simulink model "ES101A_DiagcMgr"  (R2013b)
settings: Solver=ode45  StartTime=0.0  StopTime=0.44  RelTol=1e-3
values from neighbouring files (symbols this model uses):
  BrdgVltg = DataDict.IpSignal    [ES101A_DiagcMgr_DataDict.m]
  DEM_CLEAR_PENDING = DataDict.Constant    [ES101A_DiagcMgr_DataDict.m]
  DEM_DTC_GROUP_ALL_DTCS = DataDict.Constant    [ES101A_DiagcMgr_DataDict.m]
  DFTAGICNTR_CNT_U08 = DataDict.Constant    [ES101A_DiagcMgr_DataDict.m]
  DIAGCMGR_NTCINFOSTSTESTFAILD_CNT_U08 = DataDict.Constant    [ES101A_DiagcMgr_DataDict.m]
  DIAGCMGR_NTCINFOSTSTESTFAILDTHISIGNCYC_CNT_U08 = DataDict.Constant    [ES101A_DiagcMgr_DataDict.m]
  DIAGCMGR_NTCINFOSTSTESTNOTCMPLTHISIGNCYC_CNT_U08 = DataDict.Constant    [ES101A_DiagcMgr_DataDict.m]
  DiagcMgrFltResp = DataDict.Calibration    [ES101A_DiagcMgr_DataDict.m]
  DiagcMgrNtcFltAry = DataDict.NVM    [ES101A_DiagcMgr_DataDict.m]
  DIAGCSTSCTRLDSHTDWNFLTPRSNT_CNT_U16 = DataDict.Constant    [ES101A_DiagcMgr_DataDict.m]
  DIAGCSTSDFTHWAG_CNT_U16 = DataDict.Constant    [ES101A_DiagcMgr_DataDict.m]
  DIAGCSTSDFTHWAGSERLCOMEXPRTVAL_CNT_U16 = DataDict.Constant    [ES101A_DiagcMgr_DataDict.m]
  DIAGCSTSDFTVEHSPD_CNT_U16 = DataDict.Constant    [ES101A_DiagcMgr_DataDict.m]
  DIAGCSTSININVAL_CNT_U16 = DataDict.Constant    [ES101A_DiagcMgr_DataDict.m]
  DIAGCSTSIVTR1INACTV_CNT_U16 = DataDict.Constant    [ES101A_DiagcMgr_DataDict.m]
  DIAGCSTSIVTR2INACTV_CNT_U16 = DataDict.Constant    [ES101A_DiagcMgr_DataDict.m]
  DIAGCSTSLIMDTPRFMNC_CNT_U16 = DataDict.Constant    [ES101A_DiagcMgr_DataDict.m]
  DIAGCSTSRAMPTOZEROFLTPRSNT_CNT_U16 = DataDict.Constant    [ES101A_DiagcMgr_DataDict.m]
  DIAGCSTSWHLIMBREJCTNDI_CNT_U16 = DataDict.Constant    [ES101A_DiagcMgr_DataDict.m]
  DTCIDXSTSFAIL_CNT_U08 = DataDict.Constant    [ES101A_DiagcMgr_DataDict.m]
  DTCIDXSTSNONTC_CNT_U08 = DataDict.Constant    [ES101A_DiagcMgr_DataDict.m]
  DTCIDXSTSNORES_CNT_U08 = DataDict.Constant    [ES101A_DiagcMgr_DataDict.m]
  DTCIDXSTSPASS_CNT_U08 = DataDict.Constant    [ES101A_DiagcMgr_DataDict.m]
  DTCIDXSTSUPDCFMD_CNT_U08 = DataDict.Constant    [ES101A_DiagcMgr_DataDict.m]
  ELECGLBPRM_IVTRCNT_CNT_U08 = DataDict.ConfigParam    [ES101A_DiagcMgr_DataDict.m]
  FLTINJ_DIAGCMGR_DIAGCSTSIVTR1INACTV = DataDict.Constant    [ES101A_DiagcMgr_DataDict.m]
  FLTINJ_DIAGCMGR_DIAGCSTSIVTR2INACTV = DataDict.Constant    [ES101A_DiagcMgr_DataDict.m]
  HwTq = DataDict.IpSignal    [ES101A_DiagcMgr_DataDict.m]
  IgnCntr = DataDict.IpSignal    [ES101A_DiagcMgr_DataDict.m]
  MAXDEBCNTRVAL_CNT_S16 = DataDict.Constant    [ES101A_DiagcMgr_DataDict.m]
  MAXRAMPRATE_ULSPERSEC_F32 = DataDict.Constant    [ES101A_DiagcMgr_DataDict.m]
  MINDEBCNTRVAL_CNT_S16 = DataDict.Constant    [ES101A_DiagcMgr_DataDict.m]
  MINRAMPRATE_ULSPERSEC_F32 = DataDict.Constant    [ES101A_DiagcMgr_DataDict.m]
  SCAMOTTQCMDTOONE_ULS_F32 = DataDict.Constant    [ES101A_DiagcMgr_DataDict.m]
  SCAMOTTQCMDTOZERO_ULS_F32 = DataDict.Constant    [ES101A_DiagcMgr_DataDict.m]
  SysSt = DataDict.IpSignal    [ES101A_DiagcMgr_DataDict.m]
  VehSpd = DataDict.IpSignal    [ES101A_DiagcMgr_DataDict.m]
undefined symbols (not defined in the file or in its folder): ActvMotTqCmdSca, ActvRampRate, AgiCntr, Dem_DTCFormatType, Dem_DTCOriginType, Dem_EventStatusType, DiagcData, DiagcMgrNtcMap, DiagcSts, DtcEnaMask, EcuT, HistNtcFltAry, MicroDiagcData, MotTq, NtcNr, NtcNrWithResd1, NtcStInfo, ProxySetNtcData, Sts, SysSt1, TOTNROFDTC_CNT_U08
libraries: simulink x151, FloatToFixd x5, NxtrNvM x4
(part 6 of 13)

== system ES101A_DiagcMgr/DiagcMgr/DiagcMgrPer2/Clear All DTCs/Call DEM & Update DtcIdxPrevSts/Dem_ClearDTC ==
  DTC : Inport
  DTCFormat : Inport  Port=2
  DTCOrigin : Inport  Port=3
  CopyRight2 : Subsystem  Description=|  mask(Copyright Information){none=on}
      | Copyright info block.                                               
      |                                                                     
      | Place copyright information at the top of every subsystem in design.
      mask prompts: none "No parameters"
      mask help: Place copyright information at the top of every subsystem in design.
      mask Display:
      | NxtrConf = 'Nexteer Confidential';
      | 
      | sys = bdroot; %handle for the current model ("system")
      | first = get_param(sys,'Created');
      | first = first(end-3:end);  %year is last four digits
      | 
      | last = get_param(sys,'LastModifiedDate');
      | if isempty(last)
      |     last = datestr(now,'yyyy');
      | else
      |     last = last(end-3:end);
      | end
      | 
      | if strcmp(first,last)
      |     fprintf('%s -- Copyright %s Nexteer',NxtrConf,first)
      | else
      |     fprintf('%s -- %s%s- %s Nexteer',NxtrConf,char(169),first,last)
      | end
  Ground : Ground
  Terminator : Terminator
  Terminator1 : Terminator
  Terminator2 : Terminator
  Return : Outport
  wires:
  DTC/1 -> Terminator/1
  DTCFormat/1 -> Terminator1/1
  DTCOrigin/1 -> Terminator2/1
  Ground/1 -> Return/1

== system ES101A_DiagcMgr/DiagcMgr/DiagcMgrPer2/Clear All DTCs/Call DEM & Update DtcIdxPrevSts/Update DtcIdxPrevSts and PrevClrDtcFlg ==
  Action Port : ActionPort  ActionType=then
  Clear All DTCs : Subsystem  TreatAsAtomicUnit=on
  CopyRight2 : Subsystem  Description=|  mask(Copyright Information){none=on}
      | Copyright info block.                                               
      |                                                                     
      | Place copyright information at the top of every subsystem in design.
      mask prompts: none "No parameters"
      mask help: Place copyright information at the top of every subsystem in design.
      mask Display:
      | NxtrConf = 'Nexteer Confidential';
      | 
      | sys = bdroot; %handle for the current model ("system")
      | first = get_param(sys,'Created');
      | first = first(end-3:end);  %year is last four digits
      | 
      | last = get_param(sys,'LastModifiedDate');
      | if isempty(last)
      |     last = datestr(now,'yyyy');
      | else
      |     last = last(end-3:end);
      | end
      | 
      | if strcmp(first,last)
      |     fprintf('%s -- Copyright %s Nexteer',NxtrConf,first)
      | else
      |     fprintf('%s -- %s%s- %s Nexteer',NxtrConf,char(169),first,last)
      | end
  Data Store Read1 : DataStoreRead  DataStoreName=ClrDiagcFlg
  Data Store Write2 : DataStoreWrite  DataStoreName=PrevClrDtcFlg
  wires:
  Data Store Read1/1 -> Data Store Write2/1

== system ES101A_DiagcMgr/DiagcMgr/DiagcMgrPer2/Normal Periodic Processing/For All DTCs/CopyRight2 ==

== system ES101A_DiagcMgr/DiagcMgr/DiagcMgrPer2/Normal Periodic Processing/For All DTCs/For Each DTC ==
  DtcIdxCurrSts : Inport
  DtcIdx : Inport  Port=2
  DtcIdxPrevSts : Inport  Port=3
  Check If DTC Status has Changed : Subsystem
  CopyRight2 : Subsystem  Description=|  mask(Copyright Information){none=on}
      | Copyright info block.                                               
      |                                                                     
      | Place copyright information at the top of every subsystem in design.
      mask prompts: none "No parameters"
      mask help: Place copyright information at the top of every subsystem in design.
      mask Display:
      | NxtrConf = 'Nexteer Confidential';
      | 
      | sys = bdroot; %handle for the current model ("system")
      | first = get_param(sys,'Created');
      | first = first(end-3:end);  %year is last four digits
      | 
      | last = get_param(sys,'LastModifiedDate');
      | if isempty(last)
      |     last = datestr(now,'yyyy');
      | else
      |     last = last(end-3:end);
      | end
      | 
      | if strcmp(first,last)
      |     fprintf('%s -- Copyright %s Nexteer',NxtrConf,first)
      | else
      |     fprintf('%s -- %s%s- %s Nexteer',NxtrConf,char(169),first,last)
      | end
  wires:
  DtcIdxCurrSts/1 -> Check If DTC Status has Changed/1(DtcIdxCurrSts)
  DtcIdx/1 -> Check If DTC Status has Changed/2(DtcIdx)
  DtcIdxPrevSts/1 -> Check If DTC Status has Changed/3(DtcIdxPrevSts)

== system ES101A_DiagcMgr/DiagcMgr/DiagcMgrPer2/Normal Periodic Processing/For All NTCs/CopyRight2 ==

== system ES101A_DiagcMgr/DiagcMgr/DiagcMgrPer2/Normal Periodic Processing/For All NTCs/For Each NTC ==
  note: SW Implementation:
      |
      | 	SW uses a switched case with ApplIdx as the input. The GetNtcInfoApplX is
      | 	called inside each of the switched case statements. Based on the application
      | 	index, the respective NtcInfoAryX is selected.
  ApplIdx : Inport
  NtcInfoIdx : Inport  Port=2
  NtcNr : Inport  Port=3
  Bus Selector2 : BusSelector  OutputSignals=Sts
  CopyRight2 : Subsystem  Description=|  mask(Copyright Information){none=on}
      | Copyright info block.                                               
      |                                                                     
      | Place copyright information at the top of every subsystem in design.
      mask prompts: none "No parameters"
      mask help: Place copyright information at the top of every subsystem in design.
      mask Display:
      | NxtrConf = 'Nexteer Confidential';
      | 
      | sys = bdroot; %handle for the current model ("system")
      | first = get_param(sys,'Created');
      | first = first(end-3:end);  %year is last four digits
      | 
      | last = get_param(sys,'LastModifiedDate');
      | if isempty(last)
      |     last = datestr(now,'yyyy');
      | else
      |     last = last(end-3:end);
      | end
      | 
      | if strcmp(first,last)
      |     fprintf('%s -- Copyright %s Nexteer',NxtrConf,first)
      | else
      |     fprintf('%s -- %s%s- %s Nexteer',NxtrConf,char(169),first,last)
      | end
  DoNothing : Subsystem  TreatAsAtomicUnit=on
  GetNtcInfoAppIX : Subsystem  TreatAsAtomicUnit=on
  Merge : Merge
  Switch Case : SwitchCase  CaseConditions={X}
  Update DTC Status : Subsystem  TreatAsAtomicUnit=on
  wires:
  NtcNr/1 -> Update DTC Status/1(NtcNr)
  GetNtcInfoAppIX/1(NtcInfo_ArgOut) -> Bus Selector2/1
  ApplIdx/1 -> Switch Case/1
  Switch Case/1 -> GetNtcInfoAppIX/Action
  NtcInfoIdx/1 -> GetNtcInfoAppIX/1(NtcInfoIdx_ArgIn)
  Switch Case/2 -> DoNothing/Action
  Merge/1 -> Update DTC Status/2(Sts)
  Bus Selector2/1 -> Merge/1  "<Sts>"
  DoNothing/1(Sts) -> Merge/2

== system ES101A_DiagcMgr/DiagcMgr/DiagcMgrPer2/Normal Periodic Processing/Initialize DtcIdxCurrSts/CopyRight2 ==

== system ES101A_DiagcMgr/DiagcMgr/DiagcMgrPwrDwn/Update NtcFltAry and HistFltAry/For Number of NTCs/Check Aging Counter ==
  NtcMapIdx : Inport
  AgiCntr : Inport  Port=2
  Sts : Inport  Port=3
  CopyRight2 : Subsystem  Description=|  mask(Copyright Information){none=on}
      | Copyright info block.                                               
      |                                                                     
      | Place copyright information at the top of every subsystem in design.
      mask prompts: none "No parameters"
      mask help: Place copyright information at the top of every subsystem in design.
      mask Display:
      | NxtrConf = 'Nexteer Confidential';
      | 
      | sys = bdroot; %handle for the current model ("system")
      | first = get_param(sys,'Created');
      | first = first(end-3:end);  %year is last four digits
      | 
      | last = get_param(sys,'LastModifiedDate');
      | if isempty(last)
      |     last = datestr(now,'yyyy');
      | else
      |     last = last(end-3:end);
      | end
      | 
      | if strcmp(first,last)
      |     fprintf('%s -- Copyright %s Nexteer',NxtrConf,first)
      | else
      |     fprintf('%s -- %s%s- %s Nexteer',NxtrConf,char(169),first,last)
      | end
  Do Nothing : Subsystem  TreatAsAtomicUnit=on
  If1 : If  IfExpression=u1 == 0  ElseIfExpressions=u1 < 64
  Update History Fault Array : Subsystem  TreatAsAtomicUnit=on
  Update NtcFltAry : Subsystem  TreatAsAtomicUnit=on
  wires:
  If1/3 -> Do Nothing/Action
  If1/2 -> Update History Fault Array/Action
  Sts/1 -> Update History Fault Array/2(Sts), Update NtcFltAry/2(Sts)
  NtcMapIdx/1 -> Update NtcFltAry/1(NtcMapIdx), Update History Fault Array/1(NtcMapIdx)
  AgiCntr/1 -> Update History Fault Array/3(AgiCntr), If1/1
  If1/1 -> Update NtcFltAry/Action

== system ES101A_DiagcMgr/DiagcMgr/DiagcMgrPwrDwn/Update NtcFltAry and HistFltAry/For Number of NTCs/CopyRight2 ==

== system ES101A_DiagcMgr/DiagcMgr/DiagcMgrPwrDwn/Update NtcFltAry and HistFltAry/For Number of NTCs/Default Case ==
  note: Note: Setting Aging Counter to 255 helps to identify that this NTC Number need not be store in the NvM.
      | Hence it is irrelevant what value of Status is sent out. Hence its value is set as 0.
  Action Port : ActionPort  ActionType=default
  Constant : Constant  Value=0  OutDataTypeStr=uint8
  Constant1 : Constant  Value=DFTAGICNTR_CNT_U08  OutDataTypeStr=uint8
  CopyRight2 : Subsystem  Description=|  mask(Copyright Information){none=on}
      | Copyright info block.                                               
      |                                                                     
      | Place copyright information at the top of every subsystem in design.
      mask prompts: none "No parameters"
      mask help: Place copyright information at the top of every subsystem in design.
      mask Display:
      | NxtrConf = 'Nexteer Confidential';
      | 
      | sys = bdroot; %handle for the current model ("system")
      | first = get_param(sys,'Created');
      | first = first(end-3:end);  %year is last four digits
      | 
      | last = get_param(sys,'LastModifiedDate');
      | if isempty(last)
      |     last = datestr(now,'yyyy');
      | else
      |     last = last(end-3:end);
      | end
      | 
      | if strcmp(first,last)
      |     fprintf('%s -- Copyright %s Nexteer',NxtrConf,first)
      | else
      |     fprintf('%s -- %s%s- %s Nexteer',NxtrConf,char(169),first,last)
      | end
  AgiCntr : Outport
  Sts : Outport  Port=2
  wires:
  Constant/1 -> Sts/1
  Constant1/1 -> AgiCntr/1

== system ES101A_DiagcMgr/DiagcMgr/DiagcMgrPwrDwn/Update NtcFltAry and HistFltAry/For Number of NTCs/GetNtcInfoAppIX ==
  NtcInfoIdx_ArgIn : Inport
  Action Port : ActionPort
  CopyRight2 : Subsystem  Description=|  mask(Copyright Information){none=on}
      | Copyright info block.                                               
      |                                                                     
      | Place copyright information at the top of every subsystem in design.
      mask prompts: none "No parameters"
      mask help: Place copyright information at the top of every subsystem in design.
      mask Display:
      | NxtrConf = 'Nexteer Confidential';
      | 
      | sys = bdroot; %handle for the current model ("system")
      | first = get_param(sys,'Created');
      | first = first(end-3:end);  %year is last four digits
      | 
      | last = get_param(sys,'LastModifiedDate');
      | if isempty(last)
      |     last = datestr(now,'yyyy');
      | else
      |     last = last(end-3:end);
      | end
      | 
      | if strcmp(first,last)
      |     fprintf('%s -- Copyright %s Nexteer',NxtrConf,first)
      | else
      |     fprintf('%s -- %s%s- %s Nexteer',NxtrConf,char(169),first,last)
      | end
  Data Store Read : DataStoreRead  DataStoreName=DiagcMgrNtcInfoX
  Selector : Selector  IndexMode=Zero-based  InputPortWidth=14  IndexOptions=Index vector (port)  Indices=[1 3]  OutputSizes=1
  NtcInfo_ArgOut : Outport
  wires:
  Data Store Read/1 -> Selector/1
  NtcInfoIdx_ArgIn/1 -> Selector/2
  Selector/1 -> NtcInfo_ArgOut/1

== system ES101A_DiagcMgr/DiagcMgr/DiagcMgrPwrDwn/While((HistFltAryTempIdx < HistFltInfoIdx) AND (NtcFltAryIdx < 20))/Increment HistFltAryTempIdx and NtcFltAryIdx/CopyRight1 ==

== system ES101A_DiagcMgr/DiagcMgr/DiagcMgrPwrDwn/While((HistFltAryTempIdx < HistFltInfoIdx) AND (NtcFltAryIdx < 20))/Update NtcFltAry/CopyRight1 ==

== system ES101A_DiagcMgr/DiagcMgr/DiagcMgrPwrDwn/While(CurrentFltIdx < TableSize[NtcFltAry])/Increment Indices/CopyRight1 ==

== system ES101A_DiagcMgr/DiagcMgr/DiagcMgrPwrDwn/While(CurrentFltIdx < TableSize[NtcFltAry])/Update NtcFltAry/CopyRight1 ==

== system ES101A_DiagcMgr/DiagcMgr/ReadNtcFltAry/Update DiagcMgrReadFltInfoAry and HistReadFltAry/For Number of NTCs/Check Aging Counter ==
  NtcMapIdx : Inport
  AgiCntr : Inport  Port=2
  Sts : Inport  Port=3
  NtcStInfo : Inport  Port=4
  CopyRight2 : Subsystem  Description=|  mask(Copyright Information){none=on}
      | Copyright info block.                                               
      |                                                                     
      | Place copyright information at the top of every subsystem in design.
      mask prompts: none "No parameters"
      mask help: Place copyright information at the top of every subsystem in design.
      mask Display:
      | NxtrConf = 'Nexteer Confidential';
      | 
      | sys = bdroot; %handle for the current model ("system")
      | first = get_param(sys,'Created');
      | first = first(end-3:end);  %year is last four digits
      | 
      | last = get_param(sys,'LastModifiedDate');
      | if isempty(last)
      |     last = datestr(now,'yyyy');
      | else
      |     last = last(end-3:end);
      | end
      | 
      | if strcmp(first,last)
      |     fprintf('%s -- Copyright %s Nexteer',NxtrConf,first)
      | else
      |     fprintf('%s -- %s%s- %s Nexteer',NxtrConf,char(169),first,last)
      | end
  Do Nothing : Subsystem  TreatAsAtomicUnit=on
  If1 : If  IfExpression=u1 == 0  ElseIfExpressions=u1 < 64
  Update History Fault Array : Subsystem  TreatAsAtomicUnit=on
  Update NtcFltAry : Subsystem  TreatAsAtomicUnit=on
  wires:
  If1/3 -> Do Nothing/Action
  If1/2 -> Update History Fault Array/Action
  Sts/1 -> Update NtcFltAry/2(NtcSts), Update History Fault Array/2(Sts)
  NtcMapIdx/1 -> Update NtcFltAry/1(NtcMapIdx), Update History Fault Array/1(NtcMapIdx)
  AgiCntr/1 -> Update History Fault Array/3(AgiCntr), If1/1
  If1/1 -> Update NtcFltAry/Action
  NtcStInfo/1 -> Update NtcFltAry/3(NtcStInfo), Update History Fault Array/4(NtcStInfo)

== system ES101A_DiagcMgr/DiagcMgr/ReadNtcFltAry/Update DiagcMgrReadFltInfoAry and HistReadFltAry/For Number of NTCs/CopyRight2 ==

== system ES101A_DiagcMgr/DiagcMgr/ReadNtcFltAry/Update DiagcMgrReadFltInfoAry and HistReadFltAry/For Number of NTCs/Default Case ==
  note: Note: Setting Aging Counter to 255 helps to identify that this NTC Number need not be store in the NvM.
      | Hence it is irrelevant what value of Status is sent out. Hence its value is set as 0.
  Action Port : ActionPort
  Constant : Constant  Value=0  OutDataTypeStr=uint8
  Constant1 : Constant  Value=DFTAGICNTR_CNT_U08  OutDataTypeStr=uint8
  Constant2 : Constant  Value=0  OutDataTypeStr=uint8
  CopyRight2 : Subsystem  Description=|  mask(Copyright Information){none=on}
      | Copyright info block.                                               
      |                                                                     
      | Place copyright information at the top of every subsystem in design.
      mask prompts: none "No parameters"
      mask help: Place copyright information at the top of every subsystem in design.
      mask Display:
      | NxtrConf = 'Nexteer Confidential';
      | 
      | sys = bdroot; %handle for the current model ("system")
      | first = get_param(sys,'Created');
      | first = first(end-3:end);  %year is last four digits
      | 
      | last = get_param(sys,'LastModifiedDate');
      | if isempty(last)
      |     last = datestr(now,'yyyy');
      | else
      |     last = last(end-3:end);
      | end
      | 
      | if strcmp(first,last)
      |     fprintf('%s -- Copyright %s Nexteer',NxtrConf,first)
      | else
      |     fprintf('%s -- %s%s- %s Nexteer',NxtrConf,char(169),first,last)
      | end
  AgiCntr : Outport
  Sts : Outport  Port=2
  NtcStInfo : Outport  Port=3
  wires:
  Constant/1 -> Sts/1
  Constant1/1 -> AgiCntr/1
  Constant2/1 -> NtcStInfo/1

== system ES101A_DiagcMgr/DiagcMgr/ReadNtcFltAry/Update DiagcMgrReadFltInfoAry and HistReadFltAry/For Number of NTCs/GetNtcInfoAppIX ==
  NtcInfoIdx_ArgIn : Inport
  Action Port : ActionPort
  CopyRight2 : Subsystem  Description=|  mask(Copyright Information){none=on}
      | Copyright info block.                                               
      |                                                                     
      | Place copyright information at the top of every subsystem in design.
      mask prompts: none "No parameters"
      mask help: Place copyright information at the top of every subsystem in design.
      mask Display:
      | NxtrConf = 'Nexteer Confidential';
      | 
      | sys = bdroot; %handle for the current model ("system")
      | first = get_param(sys,'Created');
      | first = first(end-3:end);  %year is last four digits
      | 
      | last = get_param(sys,'LastModifiedDate');
      | if isempty(last)
      |     last = datestr(now,'yyyy');
      | else
      |     last = last(end-3:end);
      | end
      | 
      | if strcmp(first,last)
      |     fprintf('%s -- Copyright %s Nexteer',NxtrConf,first)
      | else
      |     fprintf('%s -- %s%s- %s Nexteer',NxtrConf,char(169),first,last)
      | end
  Data Store Read : DataStoreRead  DataStoreName=DiagcMgrNtcInfoX
  Selector : Selector  IndexMode=Zero-based  InputPortWidth=14  IndexOptions=Index vector (port)  Indices=[1 3]  OutputSizes=1
  NtcInfo_ArgOut : Outport
  wires:
  Data Store Read/1 -> Selector/1
  NtcInfoIdx_ArgIn/1 -> Selector/2
  Selector/1 -> NtcInfo_ArgOut/1

== system ES101A_DiagcMgr/DiagcMgr/ReadNtcFltAry/While((HistReadFltAryTempIdx < HistReadFltAryIdx) AND (ReadFltInfoIndx < 20))/Increment HistFltAryTempdx and NtcFltAryIdx/CopyRight1 ==

== system ES101A_DiagcMgr/DiagcMgr/ReadNtcFltAry/While((HistReadFltAryTempIdx < HistReadFltAryIdx) AND (ReadFltInfoIndx < 20))/Update NtcFltAry/CopyRight1 ==

== system ES101A_DiagcMgr/DiagcMgr/ReadNtcFltAry/While(ReadFltInfoIdx < TableSize[DiagcMgrReadFltInfoAry])/Increment Indices/CopyRight1 ==

== system ES101A_DiagcMgr/DiagcMgr/ReadNtcFltAry/While(ReadFltInfoIdx < TableSize[DiagcMgrReadFltInfoAry])/Update NtcFltAry/CopyRight1 ==

== system ES101A_DiagcMgr/DiagcMgr/ReadNtcInfoAndDebCntr/ApplX/Debounced/CopyRight2 ==

== system ES101A_DiagcMgr/DiagcMgr/ReadNtcInfoAndDebCntr/ApplX/Debounced/GetNtcDebCntrApplX ==
  DebCntrIdx_ArgIn : Inport
  CopyRight2 : Subsystem  Description=|  mask(Copyright Information){none=on}
      | Copyright info block.                                               
      |                                                                     
      | Place copyright information at the top of every subsystem in design.
      mask prompts: none "No parameters"
      mask help: Place copyright information at the top of every subsystem in design.
      mask Display:
      | NxtrConf = 'Nexteer Confidential';
      | 
      | sys = bdroot; %handle for the current model ("system")
      | first = get_param(sys,'Created');
      | first = first(end-3:end);  %year is last four digits
      | 
      | last = get_param(sys,'LastModifiedDate');
      | if isempty(last)
      |     last = datestr(now,'yyyy');
      | else
      |     last = last(end-3:end);
      | end
      | 
      | if strcmp(first,last)
      |     fprintf('%s -- Copyright %s Nexteer',NxtrConf,first)
      | else
      |     fprintf('%s -- %s%s- %s Nexteer',NxtrConf,char(169),first,last)
      | end
  Data Store Read4 : DataStoreRead  DataStoreName=DiagcMgrNtcInfoXDebCntrAry
  Selector : Selector  IndexMode=Zero-based  InputPortWidth=14  IndexOptions=Index vector (port)  Indices=[1 3]  OutputSizes=1
  DebCntr_ArgOut : Outport
  wires:
  Data Store Read4/1 -> Selector/1
  DebCntrIdx_ArgIn/1 -> Selector/2
  Selector/1 -> DebCntr_ArgOut/1

== system ES101A_DiagcMgr/DiagcMgr/ReadNtcInfoAndDebCntr/ApplX/GetNtcInfoAppIX/CopyRight2 ==

== system ES101A_DiagcMgr/DiagcMgr/ReadNtcInfoAndDebCntr/ApplX/NonDebounced/CopyRight2 ==

== system ES101A_DiagcMgr/DiagcMgr/SetNtcStsCore/NtcNr is Valid/Diagnostics Inhibited/CopyRight2 ==

== system ES101A_DiagcMgr/DiagcMgr/SetNtcStsCore/NtcNr is Valid/Diagnostics Not Inhibited/CopyRight2 ==

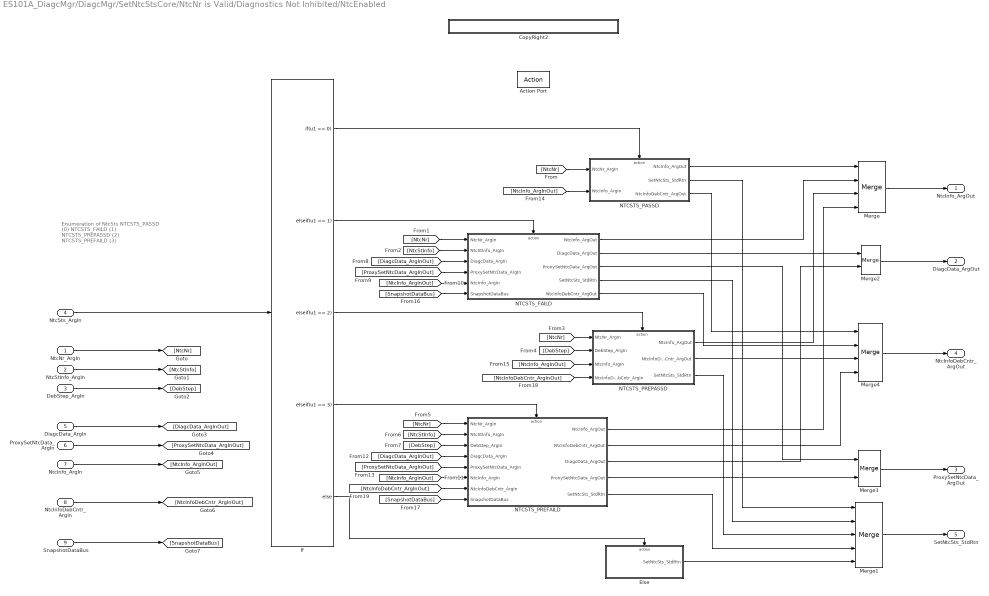
== system ES101A_DiagcMgr/DiagcMgr/SetNtcStsCore/NtcNr is Valid/Diagnostics Not Inhibited/NtcEnabled ==
  note: Enumeration of NtcSts
      |         NTCSTS_PASSD      		(0)
      |         NTCSTS_FAILD      		(1)
      |         NTCSTS_PREPASSD      	(2)
      |         NTCSTS_PREFAILD      	(3)
  NtcNr_ArgIn : Inport
  NtcStInfo_ArgIn : Inport  Port=2
  DebStep_ArgIn : Inport  Port=3
  NtcSts_ArgIn : Inport  Port=4
  DiagcData_ArgIn : Inport  Port=5
  ProxySetNtcData_ArgIn : Inport  Port=6
  NtcInfo_ArgIn : Inport  Port=7
  NtcInfoDebCntr_ArgIn : Inport  Port=8
  SnapshotDataBus : Inport  Port=9
  Action Port : ActionPort  ActionType=then
  CopyRight2 : Subsystem  Description=|  mask(Copyright Information){none=on}
      | Copyright info block.                                               
      |                                                                     
      | Place copyright information at the top of every subsystem in design.
      mask prompts: none "No parameters"
      mask help: Place copyright information at the top of every subsystem in design.
      mask Display:
      | NxtrConf = 'Nexteer Confidential';
      | 
      | sys = bdroot; %handle for the current model ("system")
      | first = get_param(sys,'Created');
      | first = first(end-3:end);  %year is last four digits
      | 
      | last = get_param(sys,'LastModifiedDate');
      | if isempty(last)
      |     last = datestr(now,'yyyy');
      | else
      |     last = last(end-3:end);
      | end
      | 
      | if strcmp(first,last)
      |     fprintf('%s -- Copyright %s Nexteer',NxtrConf,first)
      | else
      |     fprintf('%s -- %s%s- %s Nexteer',NxtrConf,char(169),first,last)
      | end
  Else : Subsystem  TreatAsAtomicUnit=on
  If : If  IfExpression=u1 == 0  ElseIfExpressions=u1 == 1, u1 == 2, u1 == 3
  Merge : Merge  Inputs=4
  Merge1 : Merge  Inputs=5
  Merge2 : Merge
  Merge3 : Merge
  Merge4 : Merge  Inputs=4
  NTCSTS_FAILD : Subsystem  TreatAsAtomicUnit=on
  NTCSTS_PASSD : Subsystem  RequirementInfo={} %GIDa_00e89d71_0d15_461b_82c5_4d6a9ccb62d4  TreatAsAtomicUnit=on
  NTCSTS_PREFAILD : Subsystem  RequirementInfo={} %GIDa_b4304517_c0d2_44f2_a1de_66f146b45b2a  TreatAsAtomicUnit=on
  NTCSTS_PREPASSD : Subsystem  RequirementInfo={} %GIDa_ee285829_c6f2_443e_92ec_6ca51b883cb1  TreatAsAtomicUnit=on
  "NtcInfo_ArgOut " : Outport
  "DiagcData_ArgOut " : Outport  Port=2
  "ProxySetNtcData_ArgOut " : Outport  Port=3
  "NtcInfoDebCntr_ArgOut " : Outport  Port=4
  SetNtcSts_StdRtn : Outport  Port=5
  wires:
  NtcSts_ArgIn/1 -> If/1
  If/1 -> NTCSTS_PASSD/Action
  If/2 -> NTCSTS_FAILD/Action
  If/3 -> NTCSTS_PREPASSD/Action
  If/4 -> NTCSTS_PREFAILD/Action
  If/5 -> Else/Action
  NtcNr_ArgIn/1 -> [NtcNr]
  NtcStInfo_ArgIn/1 -> [NtcStInfo]
  DebStep_ArgIn/1 -> [DebStep]
  [NtcNr] -> NTCSTS_PASSD/1(NtcNr_ArgIn)
  [NtcNr] -> NTCSTS_FAILD/1(NtcNr_ArgIn)
  [NtcStInfo] -> NTCSTS_FAILD/2(NtcStInfo_ArgIn)
  [NtcNr] -> NTCSTS_PREPASSD/1(NtcNr_ArgIn)
  [DebStep] -> NTCSTS_PREPASSD/2(DebStep_ArgIn)
  [NtcNr] -> NTCSTS_PREFAILD/1(NtcNr_ArgIn)
  [NtcStInfo] -> NTCSTS_PREFAILD/2(NtcStInfo_ArgIn)
  [DebStep] -> NTCSTS_PREFAILD/3(DebStep_ArgIn)
  NTCSTS_PASSD/1("NtcInfo_ArgOut ") -> Merge/1
  Merge/1 -> "NtcInfo_ArgOut "/1
  NTCSTS_FAILD/1(NtcInfo_ArgOut) -> Merge/2
  NTCSTS_PREPASSD/1(NtcInfo_ArgOut) -> Merge/3
  NTCSTS_PREFAILD/1(NtcInfo_ArgOut) -> Merge/4
  Merge1/1 -> SetNtcSts_StdRtn/1
  Else/1(SetNtcSts_StdRtn) -> Merge1/5
  NTCSTS_PREPASSD/3(SetNtcSts_StdRtn) -> Merge1/3
  NTCSTS_PREFAILD/5(SetNtcSts_StdRtn) -> Merge1/4
  NTCSTS_PASSD/2(SetNtcSts_StdRtn) -> Merge1/1
  NTCSTS_FAILD/4(SetNtcSts_StdRtn) -> Merge1/2
  DiagcData_ArgIn/1 -> [DiagcData_ArgInOut]
  ProxySetNtcData_ArgIn/1 -> [ProxySetNtcData_ArgInOut]
  NtcInfo_ArgIn/1 -> [NtcInfo_ArgInOut]
  [DiagcData_ArgInOut] -> NTCSTS_FAILD/3(DiagcData_ArgIn)
  [ProxySetNtcData_ArgInOut] -> NTCSTS_FAILD/4(ProxySetNtcData_ArgIn)
  [NtcInfo_ArgInOut] -> NTCSTS_FAILD/5(NtcInfo_ArgIn)
  [NtcInfo_ArgInOut] -> NTCSTS_PREFAILD/6(NtcInfo_ArgIn)
  [ProxySetNtcData_ArgInOut] -> NTCSTS_PREFAILD/5(ProxySetNtcData_ArgIn)
  [DiagcData_ArgInOut] -> NTCSTS_PREFAILD/4(DiagcData_ArgIn)
  [NtcInfo_ArgInOut] -> NTCSTS_PASSD/2(NtcInfo_ArgIn)
  [NtcInfo_ArgInOut] -> NTCSTS_PREPASSD/3(NtcInfo_ArgIn)
  Merge3/1 -> "ProxySetNtcData_ArgOut "/1
  Merge2/1 -> "DiagcData_ArgOut "/1
  NTCSTS_FAILD/2(DiagcData_ArgOut) -> Merge2/1
  NTCSTS_FAILD/3(ProxySetNtcData_ArgOut) -> Merge3/1
  NTCSTS_PREFAILD/3(DiagcData_ArgOut) -> Merge2/2
  NTCSTS_PREFAILD/4(ProxySetNtcData_ArgOut) -> Merge3/2
  [NtcInfoDebCntr_ArgInOut] -> NTCSTS_PREPASSD/4(NtcInfoDebCntr_ArgIn)
  [NtcInfoDebCntr_ArgInOut] -> NTCSTS_PREFAILD/7(NtcInfoDebCntr_ArgIn)
  NTCSTS_PREPASSD/2(NtcInfoDebCntr_ArgOut) -> Merge4/3
  NTCSTS_PREFAILD/2(NtcInfoDebCntr_ArgOut) -> Merge4/4
  Merge4/1 -> "NtcInfoDebCntr_ArgOut "/1
  SnapshotDataBus/1 -> [SnapshotDataBus]
  [SnapshotDataBus] -> NTCSTS_FAILD/6(SnapshotDataBus)
  [SnapshotDataBus] -> NTCSTS_PREFAILD/8(SnapshotDataBus)
  NtcInfoDebCntr_ArgIn/1 -> [NtcInfoDebCntr_ArgInOut]
  NTCSTS_PASSD/3(NtcInfoDebCntr_ArgOut) -> Merge4/1
  NTCSTS_FAILD/5(NtcInfoDebCntr_ArgOut) -> Merge4/2

== system ES101A_DiagcMgr/DiagcMgr/SetNtcStsCore/NtcNr is Valid/Diagnostics Not Inhibited/NtcNotEnabled ==
  Action Port : ActionPort  ActionType=else
  CopyRight2 : Subsystem  Description=|  mask(Copyright Information){none=on}
      | Copyright info block.                                               
      |                                                                     
      | Place copyright information at the top of every subsystem in design.
      mask prompts: none "No parameters"
      mask help: Place copyright information at the top of every subsystem in design.
      mask Display:
      | NxtrConf = 'Nexteer Confidential';
      | 
      | sys = bdroot; %handle for the current model ("system")
      | first = get_param(sys,'Created');
      | first = first(end-3:end);  %year is last four digits
      | 
      | last = get_param(sys,'LastModifiedDate');
      | if isempty(last)
      |     last = datestr(now,'yyyy');
      | else
      |     last = last(end-3:end);
      | end
      | 
      | if strcmp(first,last)
      |     fprintf('%s -- Copyright %s Nexteer',NxtrConf,first)
      | else
      |     fprintf('%s -- %s%s- %s Nexteer',NxtrConf,char(169),first,last)
      | end
  E_OK : Constant  Value=0  OutDataTypeStr=uint8
  SetNtcSts_StdRtn : Outport
  wires:
  E_OK/1 -> SetNtcSts_StdRtn/1

== system ES101A_DiagcMgr/DiagcMgr/SetNtcStsCore/NtcNr is Valid/Ntc Freeze Condition/CopyRight2 ==

== system ES101A_DiagcMgr/DiagcMgr/DiagcMgrIninCore/Initialize the NtcInfo Array/Update the ISO bits of each NTC/Start Initialization/CopyRight2 ==

== system ES101A_DiagcMgr/DiagcMgr/DiagcMgrIninCore/Initialize the NtcInfo Array/Update the ISO bits of each NTC/Start Initialization/If Action Subsystem ==
  AgiCntr : Inport
  Sts : Inport  Port=2
  Action Port : ActionPort  ActionType=else
  Clear: DIAGCMGR_NTCINFOSTSTESTFAILDTHISIGNCYC_CNT_U08 : Subsystem
  Constant1 : Constant  Value=DIAGCMGR_NTCINFOSTSTESTFAILDTHISIGNCYC_CNT_U08
  CopyRight2 : Subsystem  Description=|  mask(Copyright Information){none=on}
      | Copyright info block.                                               
      |                                                                     
      | Place copyright information at the top of every subsystem in design.
      mask prompts: none "No parameters"
      mask help: Place copyright information at the top of every subsystem in design.
      mask Display:
      | NxtrConf = 'Nexteer Confidential';
      | 
      | sys = bdroot; %handle for the current model ("system")
      | first = get_param(sys,'Created');
      | first = first(end-3:end);  %year is last four digits
      | 
      | last = get_param(sys,'LastModifiedDate');
      | if isempty(last)
      |     last = datestr(now,'yyyy');
      | else
      |     last = last(end-3:end);
      | end
      | 
      | if strcmp(first,last)
      |     fprintf('%s -- Copyright %s Nexteer',NxtrConf,first)
      | else
      |     fprintf('%s -- %s%s- %s Nexteer',NxtrConf,char(169),first,last)
      | end
  "AgiCntr " : Outport
  "Sts " : Outport  Port=2
  wires:
  AgiCntr/1 -> "AgiCntr "/1
  Constant1/1 -> Clear: DIAGCMGR_NTCINFOSTSTESTFAILDTHISIGNCYC_CNT_U08/2(In1)
  Sts/1 -> Clear: DIAGCMGR_NTCINFOSTSTESTFAILDTHISIGNCYC_CNT_U08/1(In2)
  Clear: DIAGCMGR_NTCINFOSTSTESTFAILDTHISIGNCYC_CNT_U08/1(Out1) -> "Sts "/1

== system ES101A_DiagcMgr/DiagcMgr/DiagcMgrIninCore/Initialize the NtcInfo Array/Update the ISO bits of each NTC/Start Initialization/If Action Subsystem1 ==
  Sts : Inport
  Action Port : ActionPort  ActionType=then
  Constant : Constant  Value=DFTAGICNTR_CNT_U08  OutDataTypeStr=uint8
  CopyRight2 : Subsystem  Description=|  mask(Copyright Information){none=on}
      | Copyright info block.                                               
      |                                                                     
      | Place copyright information at the top of every subsystem in design.
      mask prompts: none "No parameters"
      mask help: Place copyright information at the top of every subsystem in design.
      mask Display:
      | NxtrConf = 'Nexteer Confidential';
      | 
      | sys = bdroot; %handle for the current model ("system")
      | first = get_param(sys,'Created');
      | first = first(end-3:end);  %year is last four digits
      | 
      | last = get_param(sys,'LastModifiedDate');
      | if isempty(last)
      |     last = datestr(now,'yyyy');
      | else
      |     last = last(end-3:end);
      | end
      | 
      | if strcmp(first,last)
      |     fprintf('%s -- Copyright %s Nexteer',NxtrConf,first)
      | else
      |     fprintf('%s -- %s%s- %s Nexteer',NxtrConf,char(169),first,last)
      | end
  AgiCntr : Outport
  "Sts " : Outport  Port=2
  wires:
  Constant/1 -> AgiCntr/1
  Sts/1 -> "Sts "/1

== system ES101A_DiagcMgr/DiagcMgr/DiagcMgrIninCore/Update NtcInfoAry From NvM/Update NtcInfoAry/Update NtcInfoAry Aging Counter And Confirmed Bit/CopyRight2 ==

== system ES101A_DiagcMgr/DiagcMgr/DiagcMgrIninCore/Update NtcInfoAry From NvM/Update NtcInfoAry/Update NtcInfoAry Aging Counter And Confirmed Bit/If Action ==
  NtcNr : Inport
  AgiCntr_ArgIn : Inport  Port=2
  Sts : Inport  Port=3
  ApplIdx : Inport  Port=4
  NtcInfoAry_ArgIn : Inport  Port=5
  Action Port : ActionPort  ActionType=then
  Bus Selector3 : BusSelector  OutputSignals=ApplIdx
  Data Store Read2 : DataStoreRead  DataStoreName=DiagcMgrNtcMap  DataStoreElements=DiagcMgrNtcMap(:)
  Data Type Conversion1 : DataTypeConversion  OutDataTypeStr=uint16
  If1 : If  NumInputs=2  IfExpression=u1 == u2  ShowElse=off
  Selector2 : Selector  IndexMode=Zero-based  InputPortWidth=512  IndexOptions=Index vector (port)  Indices=[1 3]  OutputSizes=1
  Subsystem : Subsystem
  NtcInfoAry_ArgOut : Outport
  wires:
  ApplIdx/1 -> If1/2
  Data Store Read2/1 -> Selector2/1
  Selector2/1 -> Bus Selector3/1
  Data Type Conversion1/1 -> Selector2/2
  Bus Selector3/1 -> If1/1  "<ApplIdx>"
  AgiCntr_ArgIn/1 -> Subsystem/1(AgiCntr_ArgIn)
  NtcNr/1 -> Data Type Conversion1/1, Subsystem/2(NtcNr)
  Sts/1 -> Subsystem/3(Sts)
  If1/1 -> Subsystem/Action
  NtcInfoAry_ArgIn/1 -> Subsystem/4(NtcInfoAry_ArgIn)
  Subsystem/1(NtcInfoAry_ArgOut) -> NtcInfoAry_ArgOut/1

== system ES101A_DiagcMgr/DiagcMgr/DiagcMgrPer2/Clear All DTCs/Call DEM & Update DtcIdxPrevSts/Dem_ClearDTC/CopyRight2 ==

== system ES101A_DiagcMgr/DiagcMgr/DiagcMgrPer2/Clear All DTCs/Call DEM & Update DtcIdxPrevSts/Update DtcIdxPrevSts and PrevClrDtcFlg/Clear All DTCs ==
  CopyRight2 : Subsystem  Description=|  mask(Copyright Information){none=on}
      | Copyright info block.                                               
      |                                                                     
      | Place copyright information at the top of every subsystem in design.
      mask prompts: none "No parameters"
      mask help: Place copyright information at the top of every subsystem in design.
      mask Display:
      | NxtrConf = 'Nexteer Confidential';
      | 
      | sys = bdroot; %handle for the current model ("system")
      | first = get_param(sys,'Created');
      | first = first(end-3:end);  %year is last four digits
      | 
      | last = get_param(sys,'LastModifiedDate');
      | if isempty(last)
      |     last = datestr(now,'yyyy');
      | else
      |     last = last(end-3:end);
      | end
      | 
      | if strcmp(first,last)
      |     fprintf('%s -- Copyright %s Nexteer',NxtrConf,first)
      | else
      |     fprintf('%s -- %s%s- %s Nexteer',NxtrConf,char(169),first,last)
      | end
  For All DTC Indices : Subsystem
  For Iterator : ForIterator  IterationLimit=TOTNROFDTC_CNT_U08
  wires:
  For Iterator/1 -> For All DTC Indices/1(DtcIdx)

== system ES101A_DiagcMgr/DiagcMgr/DiagcMgrPer2/Clear All DTCs/Call DEM & Update DtcIdxPrevSts/Update DtcIdxPrevSts and PrevClrDtcFlg/CopyRight2 ==

== system ES101A_DiagcMgr/DiagcMgr/DiagcMgrPer2/Normal Periodic Processing/For All DTCs/For Each DTC/Check If DTC Status has Changed ==
  DtcIdxCurrSts : Inport
  DtcIdx : Inport  Port=2
  DtcIdxPrevSts : Inport  Port=3
  Bitwise Operator : simulink/Logic and Bit Operations/Bitwise Operator  logicop=AND  UseBitMask=on  BitMask=bin2dec('00000011')  BitMaskRealWorld=Stored Integer
  Bitwise Operator1 : simulink/Logic and Bit Operations/Bitwise Operator  logicop=AND  UseBitMask=on  BitMask=DTCIDXSTSUPDCFMD_CNT_U08  BitMaskRealWorld=Stored Integer
  CopyRight2 : Subsystem  Description=|  mask(Copyright Information){none=on}
      | Copyright info block.                                               
      |                                                                     
      | Place copyright information at the top of every subsystem in design.
      mask prompts: none "No parameters"
      mask help: Place copyright information at the top of every subsystem in design.
      mask Display:
      | NxtrConf = 'Nexteer Confidential';
      | 
      | sys = bdroot; %handle for the current model ("system")
      | first = get_param(sys,'Created');
      | first = first(end-3:end);  %year is last four digits
      | 
      | last = get_param(sys,'LastModifiedDate');
      | if isempty(last)
      |     last = datestr(now,'yyyy');
      | else
      |     last = last(end-3:end);
      | end
      | 
      | if strcmp(first,last)
      |     fprintf('%s -- Copyright %s Nexteer',NxtrConf,first)
      | else
      |     fprintf('%s -- %s%s- %s Nexteer',NxtrConf,char(169),first,last)
      | end
  DTC Status Changed OR DTC Update NOT Confirmed : Subsystem  TreatAsAtomicUnit=on
  Data Type Conversion : DataTypeConversion  OutDataTypeStr=uint8
  If : If  NumInputs=3  IfExpression=(u1 ~= u2) | (u3 == 0)  ShowElse=off
  wires:
  DtcIdx/1 -> DTC Status Changed OR DTC Update NOT Confirmed/1(DtcIdx)
  DtcIdxCurrSts/1 -> Data Type Conversion/1
  If/1 -> DTC Status Changed OR DTC Update NOT Confirmed/Action
  Bitwise Operator/1 -> If/2
  Data Type Conversion/1 -> If/1
  DtcIdxPrevSts/1 -> Bitwise Operator/1, Bitwise Operator1/1
  Bitwise Operator1/1 -> If/3

== system ES101A_DiagcMgr/DiagcMgr/DiagcMgrPer2/Normal Periodic Processing/For All DTCs/For Each DTC/CopyRight2 ==

== system ES101A_DiagcMgr/DiagcMgr/DiagcMgrPer2/Normal Periodic Processing/For All NTCs/For Each NTC/CopyRight2 ==

== system ES101A_DiagcMgr/DiagcMgr/DiagcMgrPer2/Normal Periodic Processing/For All NTCs/For Each NTC/DoNothing ==
  Action Port : ActionPort
  Constant : Constant  Value=DIAGCMGR_NTCINFOSTSTESTNOTCMPLTHISIGNCYC_CNT_U08  OutDataTypeStr=uint8
  CopyRight2 : Subsystem  Description=|  mask(Copyright Information){none=on}
      | Copyright info block.                                               
      |                                                                     
      | Place copyright information at the top of every subsystem in design.
      mask prompts: none "No parameters"
      mask help: Place copyright information at the top of every subsystem in design.
      mask Display:
      | NxtrConf = 'Nexteer Confidential';
      | 
      | sys = bdroot; %handle for the current model ("system")
      | first = get_param(sys,'Created');
      | first = first(end-3:end);  %year is last four digits
      | 
      | last = get_param(sys,'LastModifiedDate');
      | if isempty(last)
      |     last = datestr(now,'yyyy');
      | else
      |     last = last(end-3:end);
      | end
      | 
      | if strcmp(first,last)
      |     fprintf('%s -- Copyright %s Nexteer',NxtrConf,first)
      | else
      |     fprintf('%s -- %s%s- %s Nexteer',NxtrConf,char(169),first,last)
      | end
  Sts : Outport
  wires:
  Constant/1 -> Sts/1

== system ES101A_DiagcMgr/DiagcMgr/DiagcMgrPer2/Normal Periodic Processing/For All NTCs/For Each NTC/GetNtcInfoAppIX ==
  NtcInfoIdx_ArgIn : Inport
  Action Port : ActionPort
  CopyRight2 : Subsystem  Description=|  mask(Copyright Information){none=on}
      | Copyright info block.                                               
      |                                                                     
      | Place copyright information at the top of every subsystem in design.
      mask prompts: none "No parameters"
      mask help: Place copyright information at the top of every subsystem in design.
      mask Display:
      | NxtrConf = 'Nexteer Confidential';
      | 
      | sys = bdroot; %handle for the current model ("system")
      | first = get_param(sys,'Created');
      | first = first(end-3:end);  %year is last four digits
      | 
      | last = get_param(sys,'LastModifiedDate');
      | if isempty(last)
      |     last = datestr(now,'yyyy');
      | else
      |     last = last(end-3:end);
      | end
      | 
      | if strcmp(first,last)
      |     fprintf('%s -- Copyright %s Nexteer',NxtrConf,first)
      | else
      |     fprintf('%s -- %s%s- %s Nexteer',NxtrConf,char(169),first,last)
      | end
  Data Store Read : DataStoreRead  DataStoreName=DiagcMgrNtcInfoX
  Selector : Selector  IndexMode=Zero-based  InputPortWidth=14  IndexOptions=Index vector (port)  Indices=[1 3]  OutputSizes=1
  NtcInfo_ArgOut : Outport
  wires:
  Data Store Read/1 -> Selector/1
  NtcInfoIdx_ArgIn/1 -> Selector/2
  Selector/1 -> NtcInfo_ArgOut/1

== system ES101A_DiagcMgr/DiagcMgr/DiagcMgrPer2/Normal Periodic Processing/For All NTCs/For Each NTC/Update DTC Status ==
  NtcNr : Inport
  Sts : Inport  Port=2
  CopyRight2 : Subsystem  Description=|  mask(Copyright Information){none=on}
      | Copyright info block.                                               
      |                                                                     
      | Place copyright information at the top of every subsystem in design.
      mask prompts: none "No parameters"
      mask help: Place copyright information at the top of every subsystem in design.
      mask Display:
      | NxtrConf = 'Nexteer Confidential';
      | 
      | sys = bdroot; %handle for the current model ("system")
      | first = get_param(sys,'Created');
      | first = first(end-3:end);  %year is last four digits
      | 
      | last = get_param(sys,'LastModifiedDate');
      | if isempty(last)
      |     last = datestr(now,'yyyy');
      | else
      |     last = last(end-3:end);
      | end
      | 
      | if strcmp(first,last)
      |     fprintf('%s -- Copyright %s Nexteer',NxtrConf,first)
      | else
      |     fprintf('%s -- %s%s- %s Nexteer',NxtrConf,char(169),first,last)
      | end
  Data Type Conversion : DataTypeConversion  OutDataTypeStr=uint16
  Data Type Conversion1 : DataTypeConversion  OutDataTypeStr=uint8
  FLTRESPDTCIDX_CNT_U32 : simulink/Logic and Bit Operations/Bitwise Operator  RequirementInfo={} %GIDa_7d6b2ef8_db44_4806_9d8f_926808d52bf7  logicop=AND  UseBitMask=on  BitMask=FLTRESPDTCIDX_CNT_U32  BitMaskRealWorld=Stored Integer
  FLTRESPNTCENAD_CNT_U32 : simulink/Logic and Bit Operations/Bitwise Operator  RequirementInfo={} %GIDa_b174e7e1_8b85_4bb8_906a_fce0fbd9f834  logicop=AND  UseBitMask=on  BitMask=FLTRESPNTCENAD_CNT_U32  BitMaskRealWorld=Stored Integer
  Fault Response Table : Constant  Value=DiagcMgrFltResp
  If : If  NumInputs=3  IfExpression=(u1 ~= 0) & (u2 ~= 0) & (u2 <= u3)
  NTC Enabled : Subsystem
  NTC Not Enabled : Subsystem  TreatAsAtomicUnit=on
  Selector : Selector  IndexMode=Zero-based  InputPortWidth=512  IndexOptions=Index vector (port)  Indices=[1 3]  OutputSizes=1
  Total Number Of DTCs : Constant  Value=TOTNROFDTC_CNT_U08
  wires:
  NtcNr/1 -> Data Type Conversion/1
  Fault Response Table/1 -> Selector/1
  Selector/1 -> FLTRESPDTCIDX_CNT_U32/1, FLTRESPNTCENAD_CNT_U32/1
  Data Type Conversion/1 -> Selector/2
  FLTRESPDTCIDX_CNT_U32/1 -> Data Type Conversion1/1
  FLTRESPNTCENAD_CNT_U32/1 -> If/1
  If/1 -> NTC Enabled/Action
  If/2 -> NTC Not Enabled/Action
  Data Type Conversion1/1 -> NTC Enabled/1(DtcIdx), If/2
  Sts/1 -> NTC Enabled/2(NtcSts)
  Total Number Of DTCs/1 -> If/3

== system ES101A_DiagcMgr/DiagcMgr/DiagcMgrPwrDwn/Update NtcFltAry and HistFltAry/For Number of NTCs/Check Aging Counter/CopyRight2 ==

== system ES101A_DiagcMgr/DiagcMgr/DiagcMgrPwrDwn/Update NtcFltAry and HistFltAry/For Number of NTCs/Check Aging Counter/Do Nothing ==
  Action Port : ActionPort
  CopyRight2 : Subsystem  Description=|  mask(Copyright Information){none=on}
      | Copyright info block.                                               
      |                                                                     
      | Place copyright information at the top of every subsystem in design.
      mask prompts: none "No parameters"
      mask help: Place copyright information at the top of every subsystem in design.
      mask Display:
      | NxtrConf = 'Nexteer Confidential';
      | 
      | sys = bdroot; %handle for the current model ("system")
      | first = get_param(sys,'Created');
      | first = first(end-3:end);  %year is last four digits
      | 
      | last = get_param(sys,'LastModifiedDate');
      | if isempty(last)
      |     last = datestr(now,'yyyy');
      | else
      |     last = last(end-3:end);
      | end
      | 
      | if strcmp(first,last)
      |     fprintf('%s -- Copyright %s Nexteer',NxtrConf,first)
      | else
      |     fprintf('%s -- %s%s- %s Nexteer',NxtrConf,char(169),first,last)
      | end

== system ES101A_DiagcMgr/DiagcMgr/DiagcMgrPwrDwn/Update NtcFltAry and HistFltAry/For Number of NTCs/Check Aging Counter/Update History Fault Array ==
  NtcMapIdx : Inport
  Sts : Inport  Port=2
  AgiCntr : Inport  Port=3
  Action Port : ActionPort
  CopyRight2 : Subsystem  Description=|  mask(Copyright Information){none=on}
      | Copyright info block.                                               
      |                                                                     
      | Place copyright information at the top of every subsystem in design.
      mask prompts: none "No parameters"
      mask help: Place copyright information at the top of every subsystem in design.
      mask Display:
      | NxtrConf = 'Nexteer Confidential';
      | 
      | sys = bdroot; %handle for the current model ("system")
      | first = get_param(sys,'Created');
      | first = first(end-3:end);  %year is last four digits
      | 
      | last = get_param(sys,'LastModifiedDate');
      | if isempty(last)
      |     last = datestr(now,'yyyy');
      | else
      |     last = last(end-3:end);
      | end
      | 
      | if strcmp(first,last)
      |     fprintf('%s -- Copyright %s Nexteer',NxtrConf,first)
      | else
      |     fprintf('%s -- %s%s- %s Nexteer',NxtrConf,char(169),first,last)
      | end
  Data Store Read3 : DataStoreRead  DataStoreName=HistFltAryIdx  DataStoreElements=HistFltAryIdx
  If : If  IfExpression=u1 < 20  ShowElse=off
  If Action Subsystem : Subsystem  TreatAsAtomicUnit=on
  wires:
  If/1 -> If Action Subsystem/Action
  Data Store Read3/1 -> If/1
  Sts/1 -> If Action Subsystem/2(Sts)
  AgiCntr/1 -> If Action Subsystem/3(AgiCntr)
  NtcMapIdx/1 -> If Action Subsystem/1(NtcMapIdx)
